simulink model "SensorFailureDetection_Harness1"  (R2023b)
settings: Solver=FixedStepDiscrete  StartTime=0.0  StopTime=15  FixedStep=.1  RelTol=1e-3
libraries: simulink x2, pil_lib x1
settings Model: Creator=MOHAMED  LastModifiedBy=MOHAMED
settings DataIOCC: OutputSaveName=mdl_out  LoggingToFile=on  LoggingFileName=mdl_out.mat
settings OptimizationCC: DefaultParameterBehavior=Inlined  UseDivisionForNetSlopeComputation=on  GainParamInheritBuiltInType=on  UseFloatMulNetSlope=on  InlineInvariantSignals=on  PassReuseOutputArgsAs=Individual arguments  ZeroExternalMemoryAtStartup=off  ZeroInternalMemoryAtStartup=off  NoFixptDivByZeroProtection=on  EfficientFloat2IntCast=on  LifeSpan=1  OptimizeBlockOrder=speed  DifferentSizesBufferReuse=on  EfficientTunableParamExpr=on
settings DebuggingCC: ParameterTunabilityLossMsg=error
settings HardwareCC: ProdLongLongMode=on
settings SFSimCC: MATLABDynamicMemAlloc=off
settings RTWCC: Description=Embedded Coder  SystemTargetFile=ert.tlc  TemplateMakefile=ert_default_tmf  PortableWordSizes=on  CreateSILPILBlock=SIL
settings CodeAppCC: ForceParamTrailComments=on  IgnoreCustomStorageClasses=off  OperatorAnnotations=on  SimulinkDataObjDesc=on  SFDataObjDesc=on  CustomSymbolStrGlobalVar=rt$N$M  CustomSymbolStrType=$N$M  CustomSymbolStrFcn=$N$M$F  CustomSymbolStrMacro=$N$M  InsertBlockDesc=on
settings ERTTargetCC: TargetLangStandard=C99 (ISO)  GenerateSampleERTMain=on  IncludeMdlTerminateFcn=off  CombineSignalStateStructs=on  SuppressErrorStatus=on  SupportAbsoluteTime=off  SupportComplex=off  OptimizeReductions=on  InlinedParameterPlacement=NonHierarchical  ERTCustomFileTemplate=example_file_process.tlc  ERTFilePackagingFormat=CompactWithDataFile

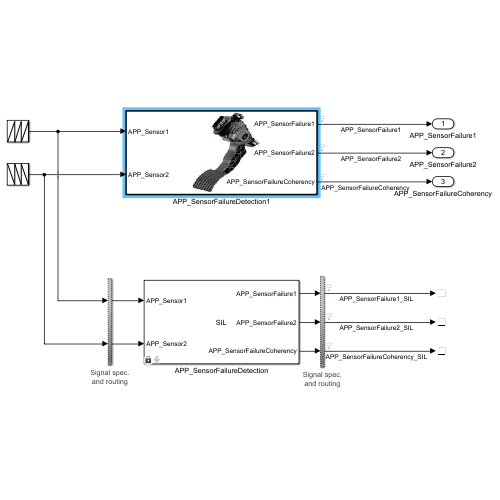
[thumbnail: Simulink's stored preview of the top-level diagram]
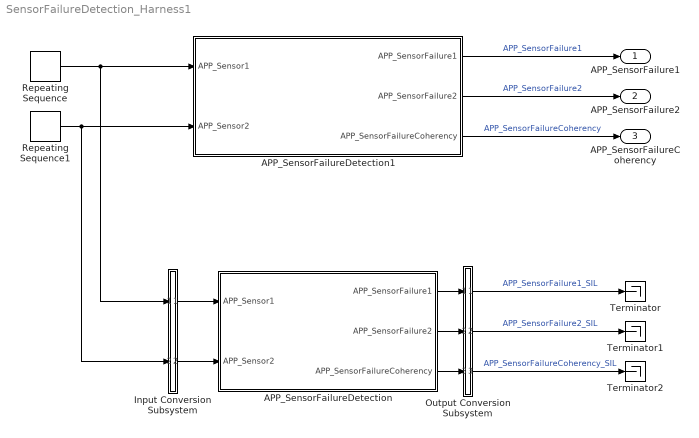
== system SensorFailureDetection_Harness1 ==
  APP_SensorFailureDetection : Subsystem  Tag=__SL_testing_harness_stub_  DialogController=pil_create_dialog  LoadFcn=|
      | try
      |    if ~strcmp(rtw.pil.getPILVersion, '23.2 (R2023b)_15')
      |       set_param(gcb, 'DialogController', '');
      |       set_param(gcb, 'DialogControllerArgs', '');
      |    end
      | catch e
      |       set_param(gcb, 'DialogController', '');
      |       set_param(gcb, 'DialogControllerArgs', '');
      | end
      mask help: PIL:pil:XILBlockMaskDesc
      mask Display: disp('SIL');
  APP_SensorFailureDetection1 : Subsystem  TreatAsAtomicUnit=on
      mask Display: image('00_Acceleration Padel Image.jpeg');
  Input Conversion Subsystem : Subsystem  Tag=__SLT_ICS__  Description=|
      | Signal spec.
      | and routing
      settings: AttributesFormatString=%<Description>
  Output Conversion Subsystem : Subsystem  Tag=__SLT_OCS__  Description=|
      | Signal spec.
      | and routing
      settings: AttributesFormatString=%<Description>
  Repeating Sequence : simulink/Sources/Repeating Sequence  rep_seq_t=[0 5]  rep_seq_y=[0 5]
  Repeating Sequence1 : simulink/Sources/Repeating Sequence  rep_seq_t=[0 4]  rep_seq_y=[5 1]
  Terminator : Terminator
  Terminator1 : Terminator
  Terminator2 : Terminator
  APP_SensorFailure1 : Outport
  APP_SensorFailure2 : Outport  Port=2
  APP_SensorFailureCoherency : Outport  Port=3
  wires:
  Output Conversion Subsystem/1(Outport_1) -> Terminator/1  "APP_SensorFailure1_SIL"
  Output Conversion Subsystem/2(Outport_2) -> Terminator1/1  "APP_SensorFailure2_SIL"
  Output Conversion Subsystem/3(Outport_3) -> Terminator2/1  "APP_SensorFailureCoherency_SIL"
  Input Conversion Subsystem/1(Outport_1) -> APP_SensorFailureDetection/1(APP_Sensor1)
  Input Conversion Subsystem/2(Outport_2) -> APP_SensorFailureDetection/2(APP_Sensor2)
  APP_SensorFailureDetection/1(APP_SensorFailure1) -> Output Conversion Subsystem/1(Inport_1)
  APP_SensorFailureDetection/2(APP_SensorFailure2) -> Output Conversion Subsystem/2(Inport_2)
  APP_SensorFailureDetection/3(APP_SensorFailureCoherency) -> Output Conversion Subsystem/3(Inport_3)
  APP_SensorFailureDetection1/2(APP_SensorFailure2) -> APP_SensorFailure2/1  "APP_SensorFailure2"
  APP_SensorFailureDetection1/1(APP_SensorFailure1) -> APP_SensorFailure1/1  "APP_SensorFailure1"
  APP_SensorFailureDetection1/3(APP_SensorFailureCoherency) -> APP_SensorFailureCoherency/1  "APP_SensorFailureCoherency"
  Repeating Sequence/1 -> Input Conversion Subsystem/1(Inport_1), APP_SensorFailureDetection1/1(APP_Sensor1)
  Repeating Sequence1/1 -> Input Conversion Subsystem/2(Inport_2), APP_SensorFailureDetection1/2(APP_Sensor2)

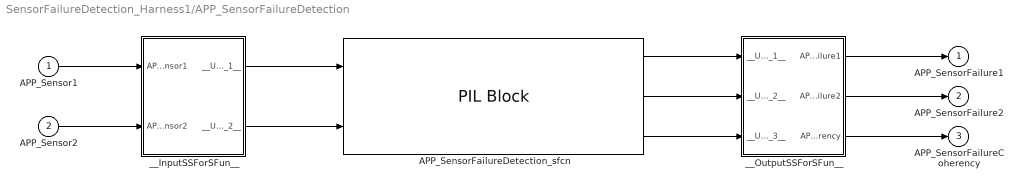
== system SensorFailureDetection_Harness1/APP_SensorFailureDetection ==
  APP_Sensor1 : Inport
  APP_Sensor2 : Inport  Port=2
  APP_SensorFailureDetection_sfcn : pil_lib/PIL Block  SimulationMode=SIL  IsTopModelPIL=off  CodeDir=APP_SensorFailureDetection_ert_rtw  AnchorDir=D:\MBD\Trail\ttt  ConfigName=Software-in-the-Loop (SIL)  XrelIsTopModelCode=on  XrelIsReusable=off  XrelDWorkNames={}  XrelDWorkTypes={}  XrelModelArgVals={}  XrelOrderedParamNames={}
  __InputSSForSFun__ : Subsystem
  __OutputSSForSFun__ : Subsystem
  APP_SensorFailure1 : Outport
  APP_SensorFailure2 : Outport  Port=2
  APP_SensorFailureCoherency : Outport  Port=3
  wires:
  __OutputSSForSFun__/3(APP_SensorFailureCoherency) -> APP_SensorFailureCoherency/1
  __OutputSSForSFun__/2(APP_SensorFailure2) -> APP_SensorFailure2/1
  __OutputSSForSFun__/1(APP_SensorFailure1) -> APP_SensorFailure1/1
  APP_SensorFailureDetection_sfcn/3 -> __OutputSSForSFun__/3(__UniqueInportName__3__)
  APP_SensorFailureDetection_sfcn/2 -> __OutputSSForSFun__/2(__UniqueInportName__2__)
  APP_SensorFailureDetection_sfcn/1 -> __OutputSSForSFun__/1(__UniqueInportName__1__)
  __InputSSForSFun__/2(__UniqueOutportName__2__) -> APP_SensorFailureDetection_sfcn/2
  __InputSSForSFun__/1(__UniqueOutportName__1__) -> APP_SensorFailureDetection_sfcn/1
  APP_Sensor2/1 -> __InputSSForSFun__/2(APP_Sensor2)
  APP_Sensor1/1 -> __InputSSForSFun__/1(APP_Sensor1)

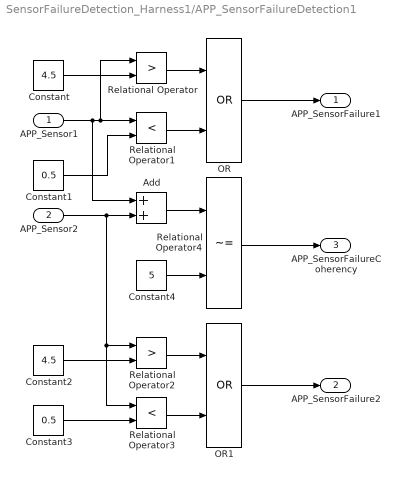
== system SensorFailureDetection_Harness1/APP_SensorFailureDetection1 ==
  APP_Sensor1 : Inport
  APP_Sensor2 : Inport  Port=2
  Add : Sum
  Constant : Constant  Value=4.5
  Constant1 : Constant  Value=0.5
  Constant2 : Constant  Value=4.5
  Constant3 : Constant  Value=0.5
  Constant4 : Constant  Value=5
  OR : Logic  Operator=OR  AllPortsSameDT=off  OutDataTypeStr=boolean
  OR1 : Logic  Operator=OR  AllPortsSameDT=off  OutDataTypeStr=boolean
  Relational Operator : RelationalOperator  Operator=>  OutDataTypeStr=boolean  RndMeth=Simplest  InputSameDT=off
  Relational Operator1 : RelationalOperator  Operator=<  OutDataTypeStr=boolean  RndMeth=Simplest  InputSameDT=off
  Relational Operator2 : RelationalOperator  Operator=>  OutDataTypeStr=boolean  RndMeth=Simplest  InputSameDT=off
  Relational Operator3 : RelationalOperator  Operator=<  OutDataTypeStr=boolean  RndMeth=Simplest  InputSameDT=off
  Relational Operator4 : RelationalOperator  Operator=~=  OutDataTypeStr=boolean  RndMeth=Simplest  InputSameDT=off
  APP_SensorFailure1 : Outport
  APP_SensorFailure2 : Outport  Port=2
  APP_SensorFailureCoherency : Outport  Port=3
  wires:
  Constant/1 -> Relational Operator/2
  Relational Operator1/1 -> OR/2
  Constant3/1 -> Relational Operator3/2
  APP_Sensor1/1 -> Relational Operator1/1, Relational Operator/1, Add/1
  Constant2/1 -> Relational Operator2/2
  APP_Sensor2/1 -> Relational Operator3/1, Relational Operator2/1, Add/2
  Constant1/1 -> Relational Operator1/2
  Relational Operator/1 -> OR/1
  Add/1 -> Relational Operator4/1
  Constant4/1 -> Relational Operator4/2
  Relational Operator2/1 -> OR1/1
  Relational Operator3/1 -> OR1/2
  OR/1 -> APP_SensorFailure1/1
  Relational Operator4/1 -> APP_SensorFailureCoherency/1
  OR1/1 -> APP_SensorFailure2/1

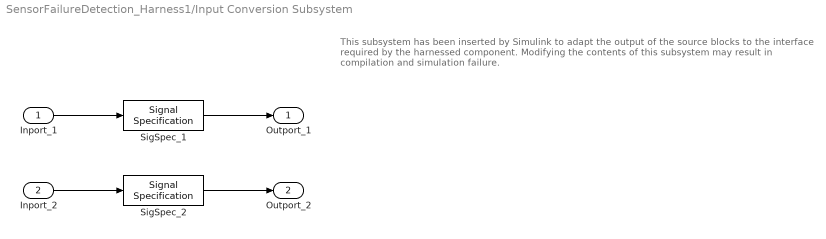
== system SensorFailureDetection_Harness1/Input Conversion Subsystem ==
  note: This subsystem has been inserted by Simulink to adapt the output of the source blocks to the interface required by the harnessed component.
      |  Modifying the contents of this subsystem may result in compilation and simulation failure.
  Inport_1 : Inport
  Inport_2 : Inport  Port=2
  SigSpec_1 : SignalSpecification  OutDataTypeStr=double  Dimensions=[1]  SampleTime=0.1
  SigSpec_2 : SignalSpecification  OutDataTypeStr=double  Dimensions=[1]  SampleTime=0.1
  Outport_1 : Outport
  Outport_2 : Outport  Port=2
  wires:
  SigSpec_1/1 -> Outport_1/1
  Inport_1/1 -> SigSpec_1/1
  SigSpec_2/1 -> Outport_2/1
  Inport_2/1 -> SigSpec_2/1

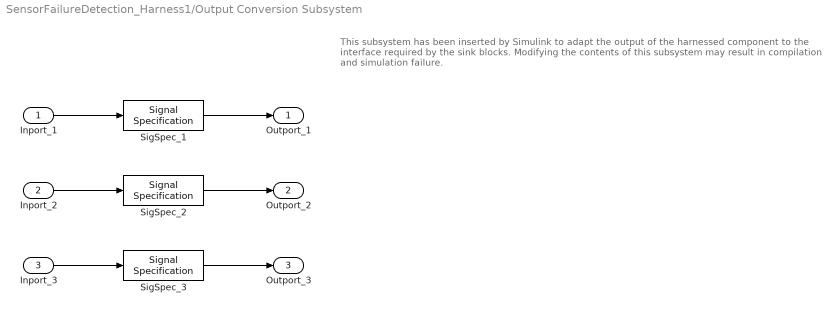
== system SensorFailureDetection_Harness1/Output Conversion Subsystem ==
  note: This subsystem has been inserted by Simulink to adapt the output of the harnessed component to the interface required by the sink blocks.
      |  Modifying the contents of this subsystem may result in compilation and simulation failure.
  Inport_1 : Inport
  Inport_2 : Inport  Port=2
  Inport_3 : Inport  Port=3
  SigSpec_1 : SignalSpecification  OutDataTypeStr=boolean  Dimensions=[1]  SampleTime=0.1
  SigSpec_2 : SignalSpecification  OutDataTypeStr=boolean  Dimensions=[1]  SampleTime=0.1
  SigSpec_3 : SignalSpecification  OutDataTypeStr=boolean  Dimensions=[1]  SampleTime=0.1
  Outport_1 : Outport
  Outport_2 : Outport  Port=2
  Outport_3 : Outport  Port=3
  wires:
  Inport_1/1 -> SigSpec_1/1
  SigSpec_1/1 -> Outport_1/1
  Inport_2/1 -> SigSpec_2/1
  SigSpec_2/1 -> Outport_2/1
  Inport_3/1 -> SigSpec_3/1
  SigSpec_3/1 -> Outport_3/1

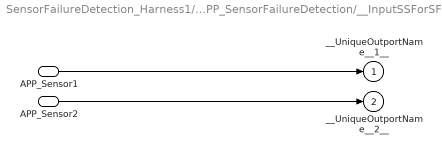
== system SensorFailureDetection_Harness1/APP_SensorFailureDetection/__InputSSForSFun__ ==
  APP_Sensor1 : Inport
  APP_Sensor2 : Inport  Port=2
  __UniqueOutportName__1__ : Outport
  __UniqueOutportName__2__ : Outport  Port=2
  wires:
  APP_Sensor2/1 -> __UniqueOutportName__2__/1
  APP_Sensor1/1 -> __UniqueOutportName__1__/1

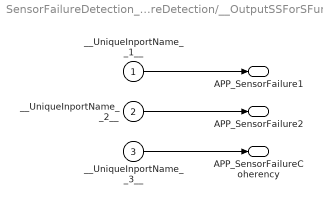
== system SensorFailureDetection_Harness1/APP_SensorFailureDetection/__OutputSSForSFun__ ==
  __UniqueInportName__1__ : Inport
  __UniqueInportName__2__ : Inport  Port=2
  __UniqueInportName__3__ : Inport  Port=3
  APP_SensorFailure1 : Outport
  APP_SensorFailure2 : Outport  Port=2
  APP_SensorFailureCoherency : Outport  Port=3
  wires:
  __UniqueInportName__3__/1 -> APP_SensorFailureCoherency/1
  __UniqueInportName__2__/1 -> APP_SensorFailure2/1
  __UniqueInportName__1__/1 -> APP_SensorFailure1/1
